simulink model "TVC_Simulink"  (R2025a)
settings: Solver=VariableStepAuto  StartTime=0.0  StopTime=5  RelTol=1e-3
libraries: slpidlib x2
settings Model: Creator=asing  LastModifiedBy=asing
settings DebuggingCC: AlgebraicLoopMsg=none

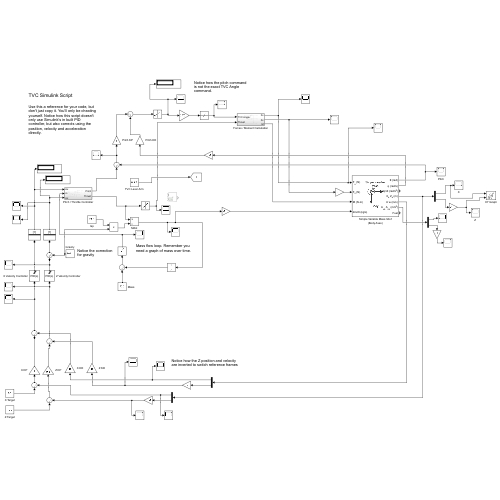
[thumbnail: Simulink's stored preview of the top-level diagram]
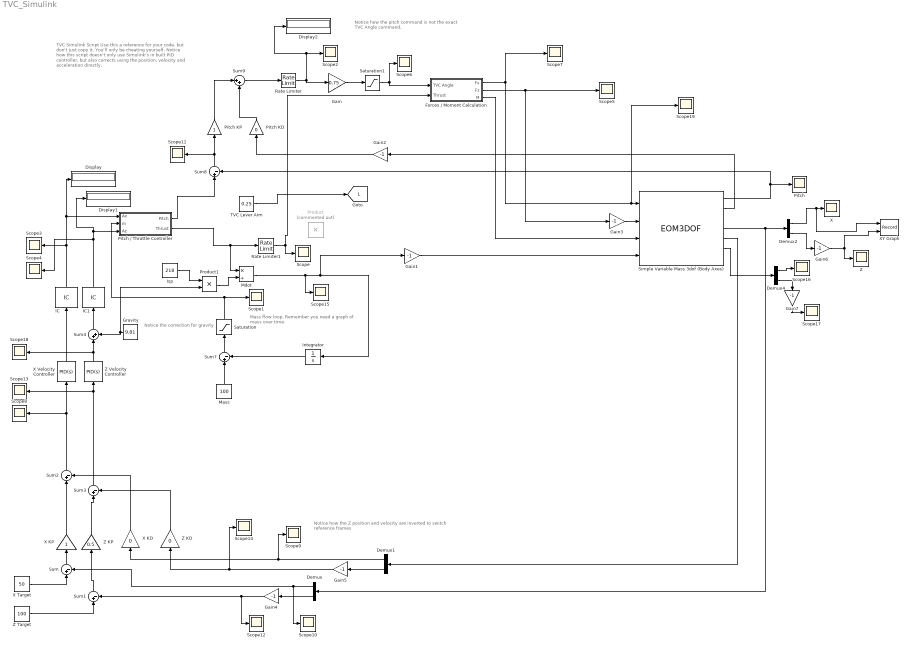
== system TVC_Simulink ==
  note: TVC Simulink Script
      |
      | Use this a reference for your code, but don't just copy it. You'll only be cheating yourself. Notice how this script doesn't only use Simulink's in built PID controller, but also corrects using the position, velocity and acceleration directly.
  note: Notice the correction for gravity
  note: Notice how the pitch command is not the exact TVC Angle command.
  note: Notice how the Z position and velocity are inverted to switch reference frames
  note: Mass flow loop. Remember you need a graph of mass over time.
  Demux{,1..2,4} (4 alike) : Demux  Outputs=2
  Display : Display
  Display1 : Display
  Display2 : Display
  Forces / Moment Calculation : Subsystem
  Gain : Gain  Gain=0.75
  Gain{1..7} (7 alike) : Gain  Gain=-1
  Gravity : Constant  Value=9.81  SampleTime=-1
  IC : InitialCondition
  IC1 : InitialCondition
  Integrator : Integrator
  Isp : Constant  Value=218  SampleTime=-1
  Mass : Constant  Value=100  SampleTime=-1
  Mdot : Product  Inputs=*/
  Pitch : Scope
      settings: ActiveDisplayYMinimum=-0.82056909143764267  ActiveDisplayYMaximum=0.0911743434930714  DataLoggingVariableName=ScopeData5
  Pitch / Throttle Controller : Subsystem
  Pitch KD : Gain  Gain=0
  Pitch KP : Gain
  Product : Product  Commented=on
  Product1 : Product
  Rate Limiter : RateLimiter  RisingSlewLimit=10  FallingSlewLimit=-inf  SampleTimeMode=inherited
  Rate Limiter1 : RateLimiter  RisingSlewLimit=50  FallingSlewLimit=-50  SampleTimeMode=inherited
  Saturation : Saturate  UpperLimit=200  LowerLimit=50
  Saturation1 : Saturate
  Scope{,1..19} (20 alike) : Scope
      Scope settings: ActiveDisplayYMinimum=2194.4088296452419  ActiveDisplayYMaximum=2422.8434633727511  DataLoggingVariableName=ScopeData2
      Scope1 settings: ActiveDisplayYMinimum=88.889157166912454  ActiveDisplayYMaximum=101.23453809256529  DataLoggingVariableName=ScopeData3
      Scope10 settings: ActiveDisplayYMinimum=-20.815065172496663  ActiveDisplayYMaximum=7.5279463716010717  DataLoggingVariableName=ScopeData14
      Scope11 settings: ActiveDisplayYMinimum=-0.954432771582435  ActiveDisplayYMaximum=1.6240869125779045  DataLoggingVariableName=ScopeData15
      Scope12 settings: ActiveDisplayYMinimum=-805.81840925124368  ActiveDisplayYMaximum=89.535378805693725  DataLoggingVariableName=ScopeData16
      Scope13 settings: ActiveDisplayYMinimum=-25.57399536801757  ActiveDisplayYMaximum=58.397110596446396  DataLoggingVariableName=ScopeData17
      Scope14 settings: ActiveDisplayYMinimum=-23.359190574528903  ActiveDisplayYMaximum=210.23271517076014  DataLoggingVariableName=ScopeData18
      Scope15 settings: ActiveDisplayYMinimum=-1  ActiveDisplayYMaximum=1  DataLoggingVariableName=ScopeData19
      Scope16 settings: DataLoggingVariableName=ScopeData20
      Scope17 settings: DataLoggingVariableName=ScopeData21
      Scope18 settings: ActiveDisplayYMinimum=-6.2499999999999982  ActiveDisplayYMaximum=56.25  DataLoggingVariableName=ScopeData22
      Scope19 settings: ActiveDisplayYMinimum=-1  ActiveDisplayYMaximum=1  DataLoggingVariableName=ScopeData23
      Scope2 settings: ActiveDisplayYMinimum=-1.2384537813656917  ActiveDisplayYMaximum=2.4582465684153676  DataLoggingVariableName=ScopeData4
      Scope3 settings: ActiveDisplayYMinimum=-12.780889310603875  ActiveDisplayYMaximum=14.853806601140857  DataLoggingVariableName=ScopeData6
      Scope4 settings: ActiveDisplayYMinimum=7.4428510639758034  ActiveDisplayYMaximum=9.9143404242177677  DataLoggingVariableName=ScopeData7
      Scope5 settings: ActiveDisplayYMinimum=226.8801933940461  ActiveDisplayYMaximum=1029.5314461063213  DataLoggingVariableName=ScopeData8
      Scope6 settings: ActiveDisplayYMinimum=-0.625  ActiveDisplayYMaximum=0.625  DataLoggingVariableName=ScopeData9
      Scope7 settings: ActiveDisplayYMinimum=-1056.9166821822043  ActiveDisplayYMaximum=1159.0366668378447  DataLoggingVariableName=ScopeData10
      Scope8 settings: ActiveDisplayYMinimum=-47.347015641611677  ActiveDisplayYMaximum=67.8668801672756  DataLoggingVariableName=ScopeData12
      Scope9 settings: ActiveDisplayYMinimum=-1  ActiveDisplayYMaximum=1  DataLoggingVariableName=ScopeData13
  Simple Variable Mass 3dof (Body Axes) : EOM3DOF  mtype=Simple Variable  v_ini=0  mass=100  mass_e=50  mass_f=100  Iyy=5000  Iyy_e=250  Iyy_f=500
  Sum{,1..3,7..8} (6 alike) : Sum  Inputs=|+-
  Sum4 : Sum  Inputs=|++
  Sum9 : Sum  Inputs=|++
  TVC Lever Arm : Constant  Value=0.25  SampleTime=-1
  X : Scope
      settings: ActiveDisplayYMinimum=-13.552881611444921  ActiveDisplayYMaximum=82.651598755514257
  X KD : Gain  Gain=0
  X KP : Gain
  X Target : Constant  Value=50  SampleTime=-1
  X Velocity Controller : slpidlib/PID Controller  Controller=PID  Form=Parallel  TimeDomain=Continuous-time  UseExternalTs=off  SampleTime=-1  IntegratorMethod=Forward Euler  FilterMethod=Forward Euler  ControllerParametersSource=internal  P=0.3  I=0  UseKiTs=off  D=0.1  UseExternalDerivativeSource=off  N=100  UseFilter=on  TunerSelectOption=Transfer Function Based (PID Tuner App)  InitialConditionSource=internal  InitialConditionForIntegrator=0  InitialConditionForFilter=0  DifferentiatorICPrevScaledInput=0  ExternalReset=none  TrackingMode=off  Kt=1  LimitOutput=on  SatLimitsSource=internal  UpperSaturationLimit=50  LowerSaturationLimit=-50  LinearizeAsGain=on  AntiWindupMode=none  Kb=1  LimitIntegrator=on  UpperIntegratorSaturationLimit=50  LowerIntegratorSaturationLimit=-50  POutMin=[]  POutMax=[]  IOutMin=[]  IOutMax=[]  DOutMin=[]  DOutMax=[]  NOutMin=[]  NOutMax=[]  SumOutMin=[]  SumOutMax=[]  SaturationOutMin=[]  SaturationOutMax=[]  PParamMin=[]  PParamMax=[]  IParamMin=[]  IParamMax=[]  DParamMin=[]  DParamMax=[]  NParamMin=[]  NParamMax=[]  KbParamMin=[]  KbParamMax=[]  KtParamMin=[]  KtParamMax=[]  KbOutMin=[]  KbOutMax=[]  KtOutMin=[]  KtOutMax=[]  IntegratorOutMin=[]  IntegratorOutMax=[]  FilterOutMin=[]  FilterOutMax=[]  SumI1OutMin=[]  SumI1OutMax=[]  SumI2OutMin=[]  SumI2OutMax=[]  SumI3OutMin=[]  SumI3OutMax=[]  SumI4OutMin=[]  SumI4OutMax=[]  SumDOutMin=[]  SumDOutMax=[]  DifferentiatorOutMin=[]  DifferentiatorOutMax=[]  FilterDiffOutCoefMin=[]  FilterDiffOutCoefMax=[]  ReciprocalOutMin=[]  ReciprocalOutMax=[]  SumDenOutMin=[]  SumDenOutMax=[]  SumNumOutMin=[]  SumNumOutMax=[]  DivideOutMin=[]  DivideOutMax=[]  UdiffTsProdOutMin=[]  UdiffTsProdOutMax=[]  NTsProdOutMin=[]  NTsProdOutMax=[]  UintegralTsProdOutMin=[]  UintegralTsProdOutMax=[]  UngainTsProdOutMin=[]  UngainTsProdOutMax=[]  ClampingZeroOutDataTypeStr=Inherit: Inherit via back propagation  ClampingZeroOutMin=[]  ClampingZeroOutMax=[]  FilterDenConstantOutDataTypeStr=Inherit: Inherit via back propagation  FilterDenConstantOutMin=[]  FilterDenConstantOutMax=[]  PCopyOutDataTypeStr=Inherit: Inherit via back propagation  PCopyOutMin=[]  PCopyOutMax=[]  NCopyOutDataTypeStr=Inherit: Inherit via back propagation  NCopyOutMin=[]  NCopyOutMax=[]  IntegratorContinuousStateAttributes=''  IntegratorStateMustResolveToSignalObject=off  IntegratorRTWStateStorageClass=Auto  FilterContinuousStateAttributes=''  FilterStateMustResolveToSignalObject=off  FilterRTWStateStorageClass=Auto  ParallelPVariant=InternalParameters  IdealPVariant=Disabled  IVariant=InternalParameters  DVariant=InternalParameters  IntegratorVariant=Continuous  SatVariant=Enabled  AWVariant=Passthrough  PCopyVariant=Disabled  TRVariant=Disabled  FdbkBlocksVariant=Forward  IdealPFdbkVariant=Disabled  SatFdbkVariant=Disabled  DerivativeFilterVariant=ContFilter  NVariant=InternalParameters  NCopyVariant=Disabled  FilterICVariant=InternalICsFilter  IntegratorICVariant=InternalICs  ExternalResetVariant=Disabled  TRSumVariant=Passthrough  SumFdbkVariant=Disabled  SumVariant=Sum_PID  TsampFilterVariant=InternalTs  TsampNgainVariant=Passthrough  TsampIntegralVariant=Disabled_SignalSpec  ExternalSaturationOutDataTypeStr=Inherit: Same as second input  DerivativeSourceVariant=ErrorSignal  PreIntVariant=InternalPreInt
  XY Graph : Record  NumPorts=2.0  FileSettingsInternal="{\"entries\":[{\"content\":{\"excelSettings\":{\"content\":{},\"type\":\"Streamout.ExcelSettings\"},\"parquetSettings\":{\"content\":{},\"type\":\"Streamout.ParquetSettings\"}},\"type\":\"Streamout.FileSettingStorage\",\"uuid\":\"\"}],\"packageUris\":[\"http:\\/\\/schema.mathworks.com\\/mf0\\/streamout_blocks\\/R2020a\"],\"version\":\"1.0\"}"  FrameSettings=[0, 0]  Layout=[1 1]  SignalsInternal="{\"entries\":[{\"content\":{\"signals\":[{\"content\":{\"blockPath\":[],\"dimensions\":[1],\"domain\":\"\",\"lineColor\":\"#a2142f\",\"plots\":[ 1 ],\"port\":1,\"signalID\":1,\"signalName\":\"Demux2:1\"},\"type\":\"RecordBlkView.Signal\",\"uuid\":\"\"},{\"content\":{\"blockPath\":[],\"dimensions\":[1],\"domain\":\"\",\"lineColor\":\"#139fff\",\"plots\":[ 1 ],\"port\":2,\"signalID\":2,\"signalName\":\"Gain6\"},\"type\":\"RecordBlkView.Signal\",\"uuid\":\"\"}]},\"type\":\"RecordBlkView.InputSignals\",\"uuid\":\"\"}],\"packageUris\":[\"http:\\/\\/schema.mathworks.com\\/mf0\\/streamout_blocks\\/R2020a\"],\"version\":\"1.0\"}"  VisualizationBindings="{\"xyplotplugin\":{\"info\":[{\"series\":[{\"bindingParametersList\":[{\"parameter\":\"X-Axis\",\"signalID\":1,\"signalName\":\"Demux2:1\"},{\"parameter\":\"Y-Axis\",\"signalID\":2,\"signalName\":\"Gain6\"}],\"seriesID\":0}],\"subplotID\":1}]}}"  CompatibilityTag=XY
  Z : Scope
      settings: ActiveDisplayYMinimum=-21.863787743348553  ActiveDisplayYMaximum=133.30722453468408
  Z KD : Gain  Gain=0
  Z KP : Gain  Gain=0.5
  Z Target : Constant  Value=100  SampleTime=-1
  Z Velocity Controller : slpidlib/PID Controller  Controller=PID  Form=Parallel  TimeDomain=Continuous-time  UseExternalTs=off  SampleTime=-1  IntegratorMethod=Forward Euler  FilterMethod=Forward Euler  ControllerParametersSource=internal  P=0.65  I=-.01  UseKiTs=off  D=0.5  UseExternalDerivativeSource=off  N=100  UseFilter=on  TunerSelectOption=Transfer Function Based (PID Tuner App)  InitialConditionSource=internal  InitialConditionForIntegrator=0  InitialConditionForFilter=0  DifferentiatorICPrevScaledInput=0  ExternalReset=none  TrackingMode=off  Kt=1  LimitOutput=on  SatLimitsSource=internal  UpperSaturationLimit=50  LowerSaturationLimit=-50  LinearizeAsGain=on  AntiWindupMode=none  Kb=1  LimitIntegrator=on  UpperIntegratorSaturationLimit=50  LowerIntegratorSaturationLimit=-50  POutMin=[]  POutMax=[]  IOutMin=[]  IOutMax=[]  DOutMin=[]  DOutMax=[]  NOutMin=[]  NOutMax=[]  SumOutMin=[]  SumOutMax=[]  SaturationOutMin=[]  SaturationOutMax=[]  PParamMin=[]  PParamMax=[]  IParamMin=[]  IParamMax=[]  DParamMin=[]  DParamMax=[]  NParamMin=[]  NParamMax=[]  KbParamMin=[]  KbParamMax=[]  KtParamMin=[]  KtParamMax=[]  KbOutMin=[]  KbOutMax=[]  KtOutMin=[]  KtOutMax=[]  IntegratorOutMin=[]  IntegratorOutMax=[]  FilterOutMin=[]  FilterOutMax=[]  SumI1OutMin=[]  SumI1OutMax=[]  SumI2OutMin=[]  SumI2OutMax=[]  SumI3OutMin=[]  SumI3OutMax=[]  SumI4OutMin=[]  SumI4OutMax=[]  SumDOutMin=[]  SumDOutMax=[]  DifferentiatorOutMin=[]  DifferentiatorOutMax=[]  FilterDiffOutCoefMin=[]  FilterDiffOutCoefMax=[]  ReciprocalOutMin=[]  ReciprocalOutMax=[]  SumDenOutMin=[]  SumDenOutMax=[]  SumNumOutMin=[]  SumNumOutMax=[]  DivideOutMin=[]  DivideOutMax=[]  UdiffTsProdOutMin=[]  UdiffTsProdOutMax=[]  NTsProdOutMin=[]  NTsProdOutMax=[]  UintegralTsProdOutMin=[]  UintegralTsProdOutMax=[]  UngainTsProdOutMin=[]  UngainTsProdOutMax=[]  ClampingZeroOutDataTypeStr=Inherit: Inherit via back propagation  ClampingZeroOutMin=[]  ClampingZeroOutMax=[]  FilterDenConstantOutDataTypeStr=Inherit: Inherit via back propagation  FilterDenConstantOutMin=[]  FilterDenConstantOutMax=[]  PCopyOutDataTypeStr=Inherit: Inherit via back propagation  PCopyOutMin=[]  PCopyOutMax=[]  NCopyOutDataTypeStr=Inherit: Inherit via back propagation  NCopyOutMin=[]  NCopyOutMax=[]  IntegratorContinuousStateAttributes=''  IntegratorStateMustResolveToSignalObject=off  IntegratorRTWStateStorageClass=Auto  FilterContinuousStateAttributes=''  FilterStateMustResolveToSignalObject=off  FilterRTWStateStorageClass=Auto  ParallelPVariant=InternalParameters  IdealPVariant=Disabled  IVariant=InternalParameters  DVariant=InternalParameters  IntegratorVariant=Continuous  SatVariant=Enabled  AWVariant=Passthrough  PCopyVariant=Disabled  TRVariant=Disabled  FdbkBlocksVariant=Forward  IdealPFdbkVariant=Disabled  SatFdbkVariant=Disabled  DerivativeFilterVariant=ContFilter  NVariant=InternalParameters  NCopyVariant=Disabled  FilterICVariant=InternalICsFilter  IntegratorICVariant=InternalICs  ExternalResetVariant=Disabled  TRSumVariant=Passthrough  SumFdbkVariant=Disabled  SumVariant=Sum_PID  TsampFilterVariant=InternalTs  TsampNgainVariant=Passthrough  TsampIntegralVariant=Disabled_SignalSpec  ExternalSaturationOutDataTypeStr=Inherit: Same as second input  DerivativeSourceVariant=ErrorSignal  PreIntVariant=InternalPreInt
  tag scope: L=global
  wires:
  Simple Variable Mass 3dof (Body Axes)/4 -> Demux2/1, Demux/1
  Simple Variable Mass 3dof (Body Axes)/5 -> Demux1/1
  X Target/1 -> Sum/1
  Z Target/1 -> Sum1/1
  Demux/1 -> Scope10/1, Sum/2
  Sum/1 -> X KP/1
  Sum1/1 -> Z KP/1
  Demux1/1 -> Scope9/1, X KD/1
  X KP/1 -> Sum2/1
  X KD/1 -> Sum2/2
  Z KD/1 -> Sum3/2
  Z KP/1 -> Sum3/1
  Sum2/1 -> Scope8/1, X Velocity Controller/1
  Sum3/1 -> Scope13/1, Z Velocity Controller/1
  X Velocity Controller/1 -> IC/1
  Gravity/1 -> Sum4/2, Product1/2
  Z Velocity Controller/1 -> Sum4/1, Scope18/1
  Sum4/1 -> IC1/1
  Mass/1 -> Sum7/1
  Integrator/1 -> Sum7/2
  Sum7/1 -> Saturation/1
  Saturation/1 -> Pitch / Throttle Controller/2(m), Scope1/1
  Simple Variable Mass 3dof (Body Axes)/1 -> Sum8/2, Pitch/1
  Simple Variable Mass 3dof (Body Axes)/2 -> Gain2/1
  Sum8/1 -> Scope11/1, Pitch KP/1
  Gain2/1 -> Pitch KD/1
  Pitch KP/1 -> Sum9/1
  Pitch KD/1 -> Sum9/2
  TVC Lever Arm/1 -> [L]
  Forces / Moment Calculation/2(Fz) -> Scope5/1, Gain3/1
  Forces / Moment Calculation/3(M) -> Simple Variable Mass 3dof (Body Axes)/3
  Demux2/1 -> XY Graph/1, X/1
  Demux2/2 -> Gain6/1
  IC/1 -> Scope3/1, Display/1, Pitch / Throttle Controller/1(Ax)
  Sum9/1 -> Rate Limiter/1
  Rate Limiter/1 -> Gain/1, Scope2/1, Display2/1
  Demux/2 -> Gain4/1
  Demux1/2 -> Gain5/1
  Pitch / Throttle Controller/1(Pitch) -> Sum8/1
  IC1/1 -> Display1/1, Pitch / Throttle Controller/3(Az), Scope4/1
  Saturation1/1 -> Forces / Moment Calculation/1(TVC Angle), Scope6/1
  Gain/1 -> Saturation1/1
  Rate Limiter1/1 -> Forces / Moment Calculation/2(Thrust), Scope/1
  Pitch / Throttle Controller/2(Thrust) -> Rate Limiter1/1, Mdot/1
  Isp/1 -> Product1/1
  Product1/1 -> Mdot/2
  Gain1/1 -> Simple Variable Mass 3dof (Body Axes)/4
  Mdot/1 -> Scope15/1, Gain1/1, Integrator/1
  Simple Variable Mass 3dof (Body Axes)/6 -> Demux4/1
  Demux4/1 -> Scope16/1
  Demux4/2 -> Gain7/1
  Gain3/1 -> Simple Variable Mass 3dof (Body Axes)/2
  Gain4/1 -> Scope12/1, Sum1/2
  Gain5/1 -> Scope14/1, Z KD/1
  Gain6/1 -> XY Graph/2, Z/1
  Gain7/1 -> Scope17/1
  Forces / Moment Calculation/1(Fx) -> Scope19/1, Simple Variable Mass 3dof (Body Axes)/1, Scope7/1

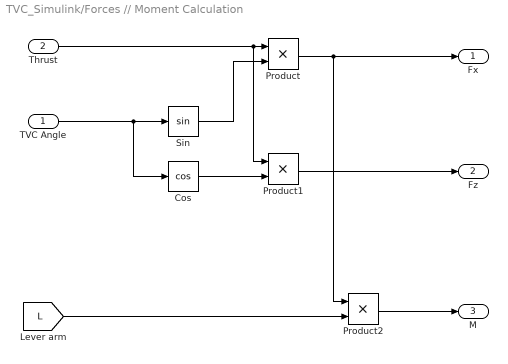
== system TVC_Simulink/Forces // Moment Calculation ==
  TVC Angle : Inport
  Thrust : Inport  Port=2
  Cos : Trigonometry  Operator=cos
  Product : Product
  Product1 : Product
  Product2 : Product
  Sin : Trigonometry
  Fx : Outport
  Fz : Outport  Port=2
  M : Outport  Port=3
  wires:
  TVC Angle/1 -> Cos/1, Sin/1
  Thrust/1 -> Product1/1, Product/1
  Sin/1 -> Product/2
  Product/1 -> Product2/1, Fx/1
  Cos/1 -> Product1/2
  Product1/1 -> Fz/1
  [L] -> Product2/2
  Product2/1 -> M/1

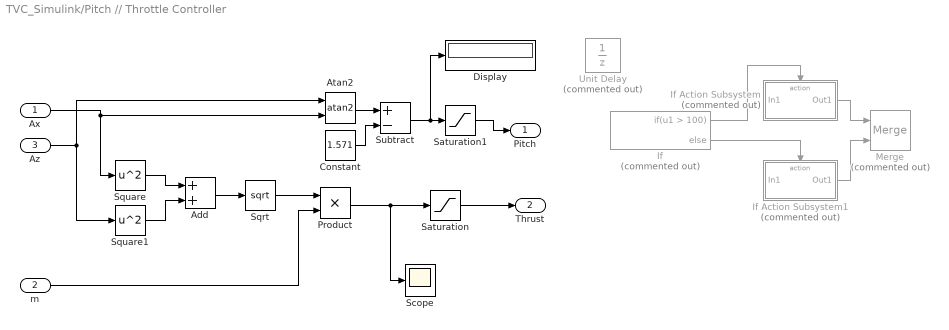
== system TVC_Simulink/Pitch // Throttle Controller ==
  Ax : Inport
  m : Inport  Port=2
  Az : Inport  Port=3
  Add : Sum
  Atan2 : Trigonometry  Operator=atan2
  Constant : Constant  Value=1.571
  Display : Display
  If : If  Commented=on  IfExpression=u1 > 100
  If Action Subsystem : Subsystem  Commented=on  TreatAsAtomicUnit=on
  If Action Subsystem1 : Subsystem  Commented=on  TreatAsAtomicUnit=on
  Merge : Merge  Commented=on
  Product : Product
  Saturation : Saturate  UpperLimit=2400  LowerLimit=890
  Saturation1 : Saturate  UpperLimit=3.14  LowerLimit=-3.14
  Scope : Scope
      settings: ActiveDisplayYMinimum=3816.6696850978651  ActiveDisplayYMaximum=10016.396600886135  DataLoggingVariableName=ScopeData11
  Sqrt : Sqrt
  Square : Math  Operator=square
  Square1 : Math  Operator=square
  Subtract : Sum  Inputs=+-
  Unit Delay : UnitDelay  Commented=on  SampleTime=-1  HasFrameUpgradeWarning=on
  Pitch : Outport
  Thrust : Outport  Port=2
  wires:
  Ax/1 -> Square/1, Atan2/2
  Az/1 -> Square1/1, Atan2/1
  m/1 -> Product/2
  Product/1 -> Scope/1, Saturation/1
  Saturation1/1 -> Pitch/1
  Square/1 -> Add/1
  Square1/1 -> Add/2
  Add/1 -> Sqrt/1
  Sqrt/1 -> Product/1
  Saturation/1 -> Thrust/1
  ? -> If Action Subsystem1/1(In1)
  If/1 -> If Action Subsystem/Action
  If/2 -> If Action Subsystem1/Action
  If Action Subsystem/1(Out1) -> Merge/1
  If Action Subsystem1/1(Out1) -> Merge/2
  Constant/1 -> Subtract/2
  Atan2/1 -> Subtract/1
  Subtract/1 -> Display/1, Saturation1/1

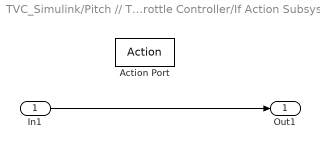
== system TVC_Simulink/Pitch // Throttle Controller/If Action Subsystem ==
  In1 : Inport
  Action Port : ActionPort  ActionPortLabel=if(u1 > 100)
  Out1 : Outport
  wires:
  In1/1 -> Out1/1

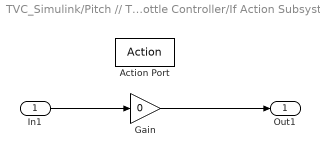
== system TVC_Simulink/Pitch // Throttle Controller/If Action Subsystem1 ==
  In1 : Inport
  Action Port : ActionPort  ActionPortLabel=else
  Gain : Gain  Gain=0
  Out1 : Outport
  wires:
  In1/1 -> Gain/1
  Gain/1 -> Out1/1
